simulink model "DE_epsIn"  (R2015a)
settings: Solver=ode15s  StartTime=0.0  StopTime=10  MaxStep=0.01  RelTol=1e-6
InitFcn:
  | Parameter;
settings Model: Creator=Johannes  LastModifiedBy=Gianluca
settings DataIOCC: SignalLoggingSaveFormat=ModelDataLogs
settings DebuggingCC: UnderspecifiedInitializationDetection=Classic  MergeDetectMultiDrivingBlocksExec=none  SolverPrmCheckMsg=warning  MultiTaskDSMMsg=warning  MultiTaskCondExecSysMsg=none  StrictBusMsg=None

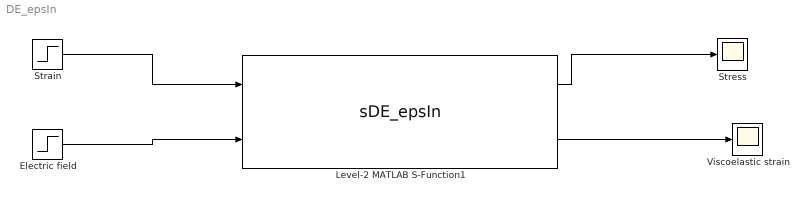
== system DE_epsIn ==
  Electric field : Step  After=0  SampleTime=0
  Level-2 MATLAB S-Function1 : M-S-Function  FunctionName=sDE_epsIn  Parameters=params, initConds
      mask Display:
      | color('black');
      | patch(4*[-1 1 1 -1],1.75*[-1 -1 1 1],[1 1 1]);
      | patch(2*[-1 1 1 -1],1.2*[-1 -1 1 1],[0 0 0]);
      | patch(1.95*[-1 1 1 -1],0.8*[-1 -1 1 1],[1 1 1]);
      | disp('DE');
      | 
      | color('blue');
      | port_label('input', 1, '\epsilon [-]','texmode','on');
      | port_label('input', 2, 'E [V/m]','texmode','on');
      | 
      | color('red');
      | port_label('output', 1, '\sigma [Pa]','texmode','on');
      | port_label('output', 2, 'x_v [-]','texmode','on');
  Strain : Step  After=0.5  SampleTime=0
  Stress : Scope
      settings: TimeRange=auto  MaxDataPoints=5000  SaveToWorkspace=off  SaveName=ScopeData  YMin=200000  YMax=1.05e+06  SampleTime=-1
  Viscoelastic strain : Scope
      settings: TimeRange=auto  MaxDataPoints=5000  SaveToWorkspace=off  YMin=0.5  YMax=0.64  SampleTime=-1
  wires:
  Strain/1 -> Level-2 MATLAB S-Function1/1
  Level-2 MATLAB S-Function1/1 -> Stress/1
  Level-2 MATLAB S-Function1/2 -> Viscoelastic strain/1
  Electric field/1 -> Level-2 MATLAB S-Function1/2
